simulink model "TrainConvoyMdl"  (R2021b)
settings: Solver=FixedStepAuto  StartTime=0.0  StopTime=500  RelTol=1e-3
undefined symbols (not defined in the file or in its folder): amax_ego, amin_ego, coupling_distance, D_default, DiscIntNeverNeededParam, t_gap, Ts, v0_ego_train_1, v0_ego_train_2, v0_lead_train, v_set, x0_ego_train_1, x0_ego_train_2, x0_lead_train
libraries: simulink x18, rllib x2
settings Model: Creator=The MathWorks, Inc.  LastModifiedBy=danif
settings SolverCC: AlgebraicLoopSolver=TrustRegion
settings DataIOCC: ReturnWorkspaceOutputs=off
settings DebuggingCC: SFMachineParentedDataDiag=warning  ArithmeticOperatorsInVariantConditions=warning
settings SFSimCC: SimUseLocalCustomCode=off
settings RTWCC: RTWUseLocalCustomCode=off
settings CodeAppCC: StateflowObjectComments=on

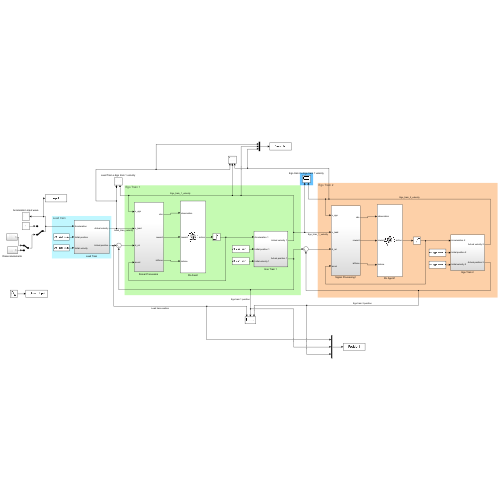
[thumbnail: Simulink's stored preview of the top-level diagram]
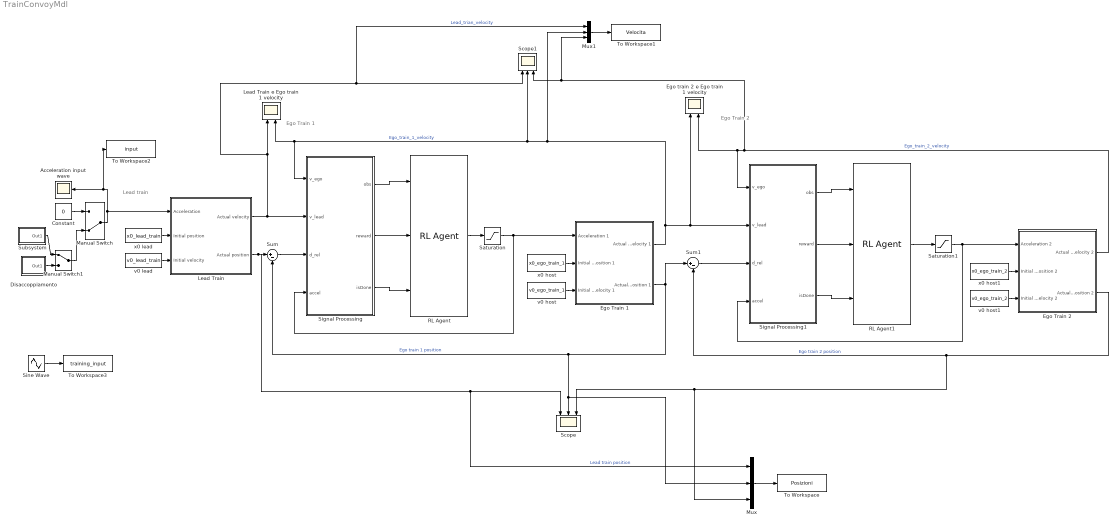
== system TrainConvoyMdl ==
  note: Lead train
  note: Ego Train 1
  note: Ego Train 2
  Acceleration input wave : Scope
  Constant : Constant  Value=0
  Disaccoppiamento : Subsystem
  Ego Train 1 : Subsystem
  Ego Train 2 : Subsystem
  Ego train 2 e Ego train 1 velocity : Scope  NumInputPorts=2
  Lead Train : Subsystem
  Lead Train e Ego train 1 velocity : Scope  NumInputPorts=2
  Manual Switch : ManualSwitch  CurrentSetting=0
  Manual Switch1 : ManualSwitch
  Mux : Mux  Inputs=3
  Mux1 : Mux  Inputs=3
  RL Agent : rllib/RL Agent  Agent=agent  ExternalActionAsInput=off  ProvideCumRwd=off  TreatAsDirectFeedthrough=on
  RL Agent1 : rllib/RL Agent  Agent=agent  ExternalActionAsInput=off  ProvideCumRwd=off  TreatAsDirectFeedthrough=on
  Saturation : Saturate  UpperLimit=amax_ego  LowerLimit=amin_ego
  Saturation1 : Saturate  UpperLimit=amax_ego  LowerLimit=amin_ego-3
  Scope : Scope  NumInputPorts=3
  Scope1 : Scope  NumInputPorts=3
  "Signal Processing " : Subsystem
  Signal Processing1 : Subsystem
  Sine Wave : Sin  Amplitude=0.6  Frequency=0.2  SampleTime=Ts
  Subsystem : Subsystem
  Sum : Sum  Inputs=|+-
  Sum1 : Sum  Inputs=|+-
  To Workspace : ToWorkspace  VariableName=Posizioni  SaveFormat=Timeseries  SampleTime=-1
  To Workspace1 : ToWorkspace  VariableName=Velocita  SaveFormat=Timeseries  SampleTime=-1
  To Workspace2 : ToWorkspace  VariableName=input  SaveFormat=Timeseries  SampleTime=-1
  To Workspace3 : ToWorkspace  VariableName=training_input  SaveFormat=Timeseries  SampleTime=-1
  v0 host : Constant  Value=v0_ego_train_1  SampleTime=Ts
  v0 host1 : Constant  Value=v0_ego_train_2  SampleTime=Ts
  v0 lead : Constant  Value=v0_lead_train  SampleTime=Ts
  x0 host : Constant  Value=x0_ego_train_1  SampleTime=Ts
  x0 host1 : Constant  Value=x0_ego_train_2  SampleTime=Ts
  x0 lead : Constant  Value=x0_lead_train  SampleTime=Ts
  wires:
  x0 lead/1 -> Lead Train/2(Initial position)
  v0 lead/1 -> Lead Train/3(Initial velocity)
  x0 host/1 -> Ego Train 1/2(Initial position 1)
  Ego Train 1/2(Actual position 1) -> Sum1/1, Sum/2, Mux/2, Scope/2  "Ego train 1 position"
  v0 host/1 -> Ego Train 1/3(Initial velocity 1)
  Lead Train/1(Actual velocity) -> "Signal Processing "/2(v_lead), Mux1/1, Scope1/1, Lead Train e Ego train 1 velocity/1  "Lead_trian_velocity"
  "Signal Processing "/2(reward) -> RL Agent/2
  Saturation/1 -> Ego Train 1/1(Acceleration 1), "Signal Processing "/4(accel)
  RL Agent/1 -> Saturation/1
  "Signal Processing "/3(isDone) -> RL Agent/3
  "Signal Processing "/1(obs) -> RL Agent/1
  Sum/1 -> "Signal Processing "/3(d_rel)
  Ego Train 1/1(Actual velocity 1) -> Signal Processing1/2(v_lead), Ego train 2 e Ego train 1 velocity/1, Mux1/2, "Signal Processing "/1(v_ego), Lead Train e Ego train 1 velocity/2, Scope1/2  "Ego_train_1_velocity"
  Ego Train 2/1(Actual velocity 2) -> Signal Processing1/1(v_ego), Ego train 2 e Ego train 1 velocity/2, Mux1/3, Scope1/3  "Ego_train_2_velocity"
  Sum1/1 -> Signal Processing1/3(d_rel)
  Signal Processing1/2(reward) -> RL Agent1/2
  Signal Processing1/1(obs) -> RL Agent1/1
  RL Agent1/1 -> Saturation1/1
  Saturation1/1 -> Ego Train 2/1(Acceleration 2), Signal Processing1/4(accel)
  Signal Processing1/3(isDone) -> RL Agent1/3
  Ego Train 2/2(Actual position 2) -> Mux/3, Scope/3, Sum1/2  "Ego train 2 position"
  v0 host1/1 -> Ego Train 2/3(Initial velocity 2)
  x0 host1/1 -> Ego Train 2/2(Initial position 2)
  Manual Switch/1 -> To Workspace2/1, Acceleration input wave/1, Lead Train/1(Acceleration)
  Constant/1 -> Manual Switch/1
  Lead Train/2(Actual position) -> Mux/1, Scope/1, Sum/1  "Lead train position"
  Disaccoppiamento/1(Out1) -> Manual Switch1/2
  Manual Switch1/1 -> Manual Switch/2
  Subsystem/1(Out1) -> Manual Switch1/1
  Mux/1 -> To Workspace/1
  Mux1/1 -> To Workspace1/1
  Sine Wave/1 -> To Workspace3/1

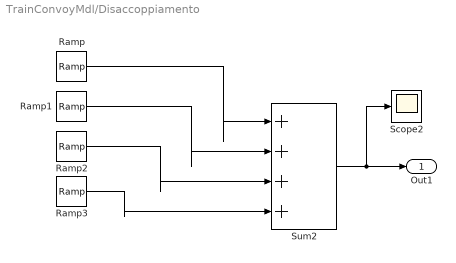
== system TrainConvoyMdl/Disaccoppiamento ==
  Ramp : simulink/Sources/Ramp  slope=0.005  start=70  InitialOutput=0
  Ramp1 : simulink/Sources/Ramp  slope=-0.005  start=130  InitialOutput=0
  Ramp2 : simulink/Sources/Ramp  slope=-0.005  start=260  InitialOutput=0
  Ramp3 : simulink/Sources/Ramp  slope=0.005  start=320  InitialOutput=0
  Scope2 : Scope
  Sum2 : Sum  Inputs=|++++
  Out1 : Outport
  wires:
  Ramp2/1 -> Sum2/3
  Sum2/1 -> Out1/1, Scope2/1
  Ramp1/1 -> Sum2/2
  Ramp3/1 -> Sum2/4
  Ramp/1 -> Sum2/1

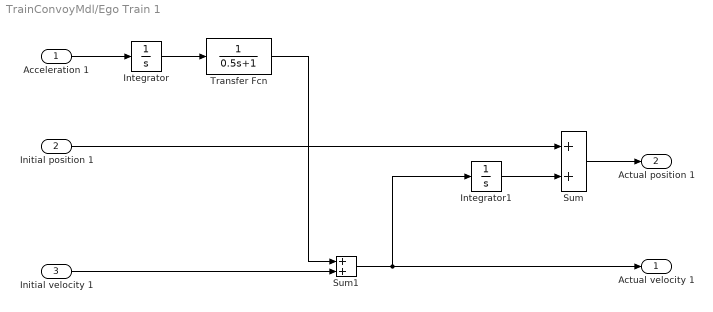
== system TrainConvoyMdl/Ego Train 1 ==
  Acceleration 1 : Inport
  Initial position 1 : Inport  Port=2
  Initial velocity 1 : Inport  Port=3
  Integrator : Integrator
  Integrator1 : Integrator
  Sum : Sum
  Sum1 : Sum
  Transfer Fcn : TransferFcn  Denominator=[0.5 1]
  Actual velocity 1 : Outport  VectorParamsAs1DForOutWhenUnconnected=off
  Actual position 1 : Outport  Port=2  VectorParamsAs1DForOutWhenUnconnected=off
  wires:
  Sum1/1 -> Integrator1/1, Actual velocity 1/1
  Initial velocity 1/1 -> Sum1/2
  Sum/1 -> Actual position 1/1
  Transfer Fcn/1 -> Sum1/1
  Integrator/1 -> Transfer Fcn/1
  Acceleration 1/1 -> Integrator/1
  Initial position 1/1 -> Sum/1
  Integrator1/1 -> Sum/2

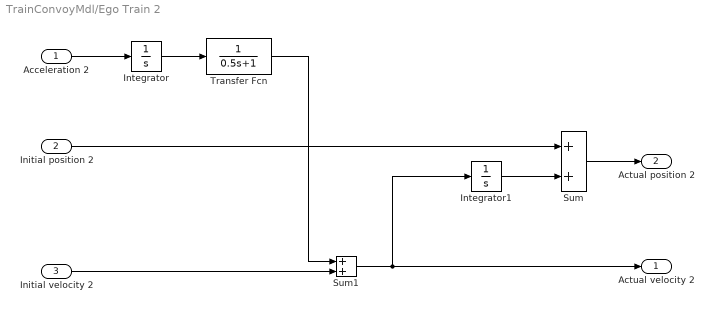
== system TrainConvoyMdl/Ego Train 2 ==
  Acceleration 2 : Inport
  Initial position 2 : Inport  Port=2
  Initial velocity 2 : Inport  Port=3
  Integrator : Integrator
  Integrator1 : Integrator
  Sum : Sum
  Sum1 : Sum
  Transfer Fcn : TransferFcn  Denominator=[0.5 1]
  Actual velocity 2 : Outport  VectorParamsAs1DForOutWhenUnconnected=off
  Actual position 2 : Outport  Port=2  VectorParamsAs1DForOutWhenUnconnected=off
  wires:
  Sum1/1 -> Integrator1/1, Actual velocity 2/1
  Initial velocity 2/1 -> Sum1/2
  Sum/1 -> Actual position 2/1
  Transfer Fcn/1 -> Sum1/1
  Integrator/1 -> Transfer Fcn/1
  Acceleration 2/1 -> Integrator/1
  Initial position 2/1 -> Sum/1
  Integrator1/1 -> Sum/2

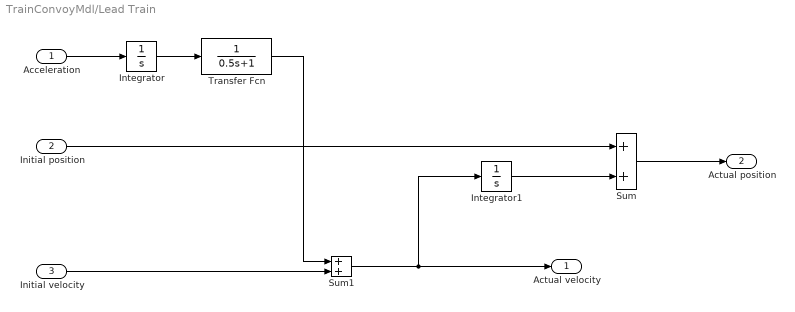
== system TrainConvoyMdl/Lead Train ==
  Acceleration : Inport
  Initial position : Inport  Port=2
  Initial velocity : Inport  Port=3
  Integrator : Integrator
  Integrator1 : Integrator
  Sum : Sum
  Sum1 : Sum
  Transfer Fcn : TransferFcn  Denominator=[0.5 1]
  Actual velocity : Outport  VectorParamsAs1DForOutWhenUnconnected=off
  Actual position : Outport  Port=2  VectorParamsAs1DForOutWhenUnconnected=off
  wires:
  Transfer Fcn/1 -> Sum1/1
  Initial velocity/1 -> Sum1/2
  Sum/1 -> Actual position/1
  Integrator/1 -> Transfer Fcn/1
  Sum1/1 -> Integrator1/1, Actual velocity/1
  Acceleration/1 -> Integrator/1
  Initial position/1 -> Sum/1
  Integrator1/1 -> Sum/2

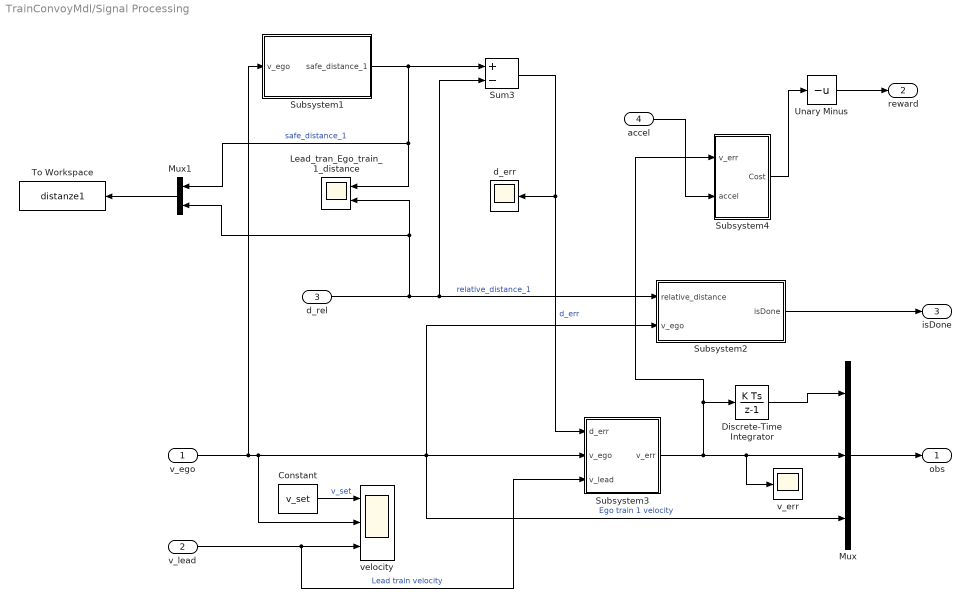
== system TrainConvoyMdl/Signal Processing  ==
  v_ego : Inport
  v_lead : Inport  Port=2
  d_rel : Inport  Port=3
  accel : Inport  Port=4
  Constant : Constant  Value=v_set
  Discrete-Time Integrator : DiscreteIntegrator  SampleTime=-1  ICPrevOutput=DiscIntNeverNeededParam  ICPrevScaledInput=DiscIntNeverNeededParam
  Lead_tran_Ego_train_1_distance : Scope  NumInputPorts=2
  Mux : Mux  Inputs=3
  Mux1 : Mux  Inputs=2
  Subsystem1 : Subsystem
  Subsystem2 : Subsystem
  Subsystem3 : Subsystem
  Subsystem4 : Subsystem
  Sum3 : Sum  Inputs=+-
  To Workspace : ToWorkspace  VariableName=distanze1  SaveFormat=Timeseries  SampleTime=-1
  Unary Minus : UnaryMinus
  d_err : Scope
  v_err : Scope
  velocity : Scope  NumInputPorts=3
  obs : Outport  VectorParamsAs1DForOutWhenUnconnected=off
  reward : Outport  Port=2  VectorParamsAs1DForOutWhenUnconnected=off
  isDone : Outport  Port=3  VectorParamsAs1DForOutWhenUnconnected=off
  wires:
  Constant/1 -> velocity/1  "v_set"
  v_lead/1 -> velocity/3, Subsystem3/3(v_lead)  "Lead train velocity"
  Mux/1 -> obs/1
  v_ego/1 -> velocity/2, Subsystem3/2(v_ego), Mux/3, Subsystem2/2(v_ego), Subsystem1/1(v_ego)  "Ego train 1 velocity"
  d_rel/1 -> Subsystem2/1(relative_distance), Sum3/2, Mux1/2, Lead_tran_Ego_train_1_distance/2  "relative_distance_1"
  Subsystem4/1(Cost) -> Unary Minus/1
  Unary Minus/1 -> reward/1
  Sum3/1 -> Subsystem3/1(d_err), d_err/1  "d_err"
  Subsystem1/1(safe_distance_1) -> Mux1/1, Lead_tran_Ego_train_1_distance/1, Sum3/1  "safe_distance_1"
  accel/1 -> Subsystem4/2(accel)
  Subsystem2/1(isDone) -> isDone/1
  Subsystem3/1(v_err) -> Subsystem4/1(v_err), Discrete-Time Integrator/1, v_err/1, Mux/2
  Discrete-Time Integrator/1 -> Mux/1
  Mux1/1 -> To Workspace/1

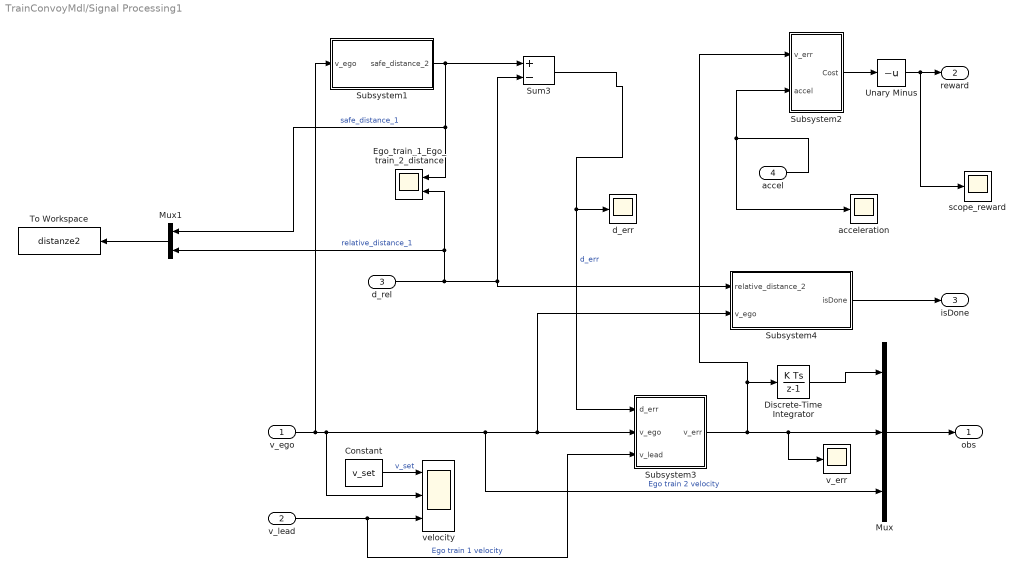
== system TrainConvoyMdl/Signal Processing1 ==
  v_ego : Inport
  v_lead : Inport  Port=2
  d_rel : Inport  Port=3
  accel : Inport  Port=4
  Constant : Constant  Value=v_set
  Discrete-Time Integrator : DiscreteIntegrator  SampleTime=-1  ICPrevOutput=DiscIntNeverNeededParam  ICPrevScaledInput=DiscIntNeverNeededParam
  Ego_train_1_Ego_train_2_distance : Scope  NumInputPorts=2
  Mux : Mux  Inputs=3
  Mux1 : Mux  Inputs=2
  Subsystem1 : Subsystem
  Subsystem2 : Subsystem
  Subsystem3 : Subsystem
  Subsystem4 : Subsystem
  Sum3 : Sum  Inputs=+-
  To Workspace : ToWorkspace  VariableName=distanze2  SaveFormat=Timeseries  SampleTime=-1
  Unary Minus : UnaryMinus
  acceleration : Scope
  d_err : Scope
  scope_reward : Scope
  v_err : Scope
  velocity : Scope  NumInputPorts=3
  obs : Outport  VectorParamsAs1DForOutWhenUnconnected=off
  reward : Outport  Port=2  VectorParamsAs1DForOutWhenUnconnected=off
  isDone : Outport  Port=3  VectorParamsAs1DForOutWhenUnconnected=off
  wires:
  Constant/1 -> velocity/1  "v_set"
  v_lead/1 -> velocity/3, Subsystem3/3(v_lead)  "Ego train 1 velocity"
  Mux/1 -> obs/1
  v_ego/1 -> velocity/2, Subsystem4/2(v_ego), Subsystem3/2(v_ego), Mux/3, Subsystem1/1(v_ego)  "Ego train 2 velocity"
  Subsystem2/1(Cost) -> Unary Minus/1
  Sum3/1 -> d_err/1, Subsystem3/1(d_err)  "d_err"
  accel/1 -> Subsystem2/2(accel), acceleration/1
  Subsystem4/1(isDone) -> isDone/1
  Subsystem3/1(v_err) -> Subsystem2/1(v_err), Discrete-Time Integrator/1, v_err/1, Mux/2
  Discrete-Time Integrator/1 -> Mux/1
  Unary Minus/1 -> scope_reward/1, reward/1
  d_rel/1 -> Subsystem4/1(relative_distance_2), Sum3/2, Ego_train_1_Ego_train_2_distance/2, Mux1/2  "relative_distance_1"
  Mux1/1 -> To Workspace/1
  Subsystem1/1(safe_distance_2) -> Mux1/1, Ego_train_1_Ego_train_2_distance/1, Sum3/1  "safe_distance_1"

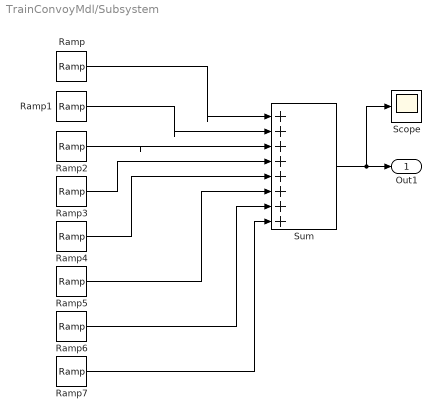
== system TrainConvoyMdl/Subsystem ==
  Ramp : simulink/Sources/Ramp  slope=0.005  start=70  InitialOutput=0
  Ramp1 : simulink/Sources/Ramp  slope=-0.005  start=110  InitialOutput=0
  Ramp2 : simulink/Sources/Ramp  slope=-0.005  start=140  InitialOutput=0
  Ramp3 : simulink/Sources/Ramp  slope=0.005  start=180  InitialOutput=0
  Ramp4 : simulink/Sources/Ramp  slope=-0.005  start=230  InitialOutput=0
  Ramp5 : simulink/Sources/Ramp  slope=0.005  start=280  InitialOutput=0
  Ramp6 : simulink/Sources/Ramp  slope=0.005  start=320  InitialOutput=0
  Ramp7 : simulink/Sources/Ramp  slope=-0.005  start=370  InitialOutput=0
  Scope : Scope
  Sum : Sum  Inputs=|++++++++
  Out1 : Outport
  wires:
  Ramp/1 -> Sum/1
  Ramp2/1 -> Sum/3
  Ramp1/1 -> Sum/2
  Ramp3/1 -> Sum/4
  Sum/1 -> Scope/1, Out1/1
  Ramp4/1 -> Sum/5
  Ramp5/1 -> Sum/6
  Ramp6/1 -> Sum/7
  Ramp7/1 -> Sum/8

== system TrainConvoyMdl/Signal Processing /Subsystem1 ==
  v_ego : Inport
  Default Spacing : Constant  Value=D_default  SampleTime=Ts
  Product : Product
  Sum2 : Sum
  Time Gap : Constant  Value=t_gap  SampleTime=Ts
  safe_distance_1 : Outport  VectorParamsAs1DForOutWhenUnconnected=off
  wires:
  Sum2/1 -> safe_distance_1/1
  Time Gap/1 -> Product/2
  Default Spacing/1 -> Sum2/1
  v_ego/1 -> Product/1
  Product/1 -> Sum2/2

== system TrainConvoyMdl/Signal Processing /Subsystem2 ==
  relative_distance : Inport
  v_ego : Inport  Port=2
  Logical Operator : Logic  Operator=OR  AllPortsSameDT=off  OutDataTypeStr=boolean
  Relative Distance : simulink/Logic and Bit Operations/Compare To Constant  relop=<  const=0  OutDataTypeStr=boolean
  Velocity : simulink/Logic and Bit Operations/Compare To Constant  relop=<  const=0  OutDataTypeStr=boolean
  isDone : Outport  VectorParamsAs1DForOutWhenUnconnected=off
  wires:
  Velocity/1 -> Logical Operator/2
  Relative Distance/1 -> Logical Operator/1
  Logical Operator/1 -> isDone/1
  v_ego/1 -> Velocity/1
  relative_distance/1 -> Relative Distance/1

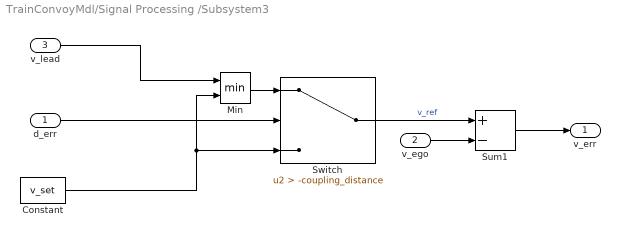
== system TrainConvoyMdl/Signal Processing /Subsystem3 ==
  d_err : Inport
  v_ego : Inport  Port=2
  v_lead : Inport  Port=3
  Constant : Constant  Value=v_set
  Min : MinMax  Inputs=2
  Sum1 : Sum  Inputs=+-
  Switch : Switch  Criteria=u2 > Threshold  Threshold=-coupling_distance
  v_err : Outport  VectorParamsAs1DForOutWhenUnconnected=off
  wires:
  Sum1/1 -> v_err/1
  v_ego/1 -> Sum1/2
  d_err/1 -> Switch/2
  Constant/1 -> Min/2, Switch/3
  Min/1 -> Switch/1
  v_lead/1 -> Min/1
  Switch/1 -> Sum1/1  "v_ref"

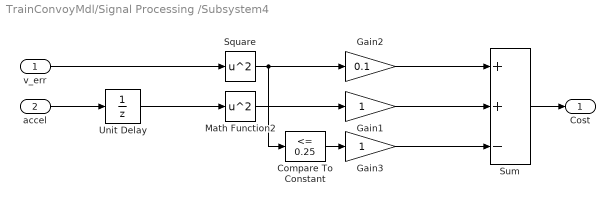
== system TrainConvoyMdl/Signal Processing /Subsystem4 ==
  v_err : Inport
  accel : Inport  Port=2
  Compare To Constant : simulink/Logic and Bit Operations/Compare To Constant  relop=<=  const=0.25  OutDataTypeStr=boolean
  Gain1 : Gain
  Gain2 : Gain  Gain=0.1
  Gain3 : Gain
  Math Function2 : Math  Operator=square  SignedPower=on  SaturateOnIntegerOverflow=on
  Square : Math  Operator=square  SignedPower=on  SaturateOnIntegerOverflow=on
  Sum : Sum  Inputs=++-
  Unit Delay : UnitDelay  SampleTime=-1  HasFrameUpgradeWarning=on
  Cost : Outport  VectorParamsAs1DForOutWhenUnconnected=off
  wires:
  v_err/1 -> Square/1
  Math Function2/1 -> Gain1/1
  accel/1 -> Unit Delay/1
  Sum/1 -> Cost/1
  Square/1 -> Compare To Constant/1, Gain2/1
  Unit Delay/1 -> Math Function2/1
  Gain2/1 -> Sum/1
  Gain1/1 -> Sum/2
  Compare To Constant/1 -> Gain3/1
  Gain3/1 -> Sum/3

== system TrainConvoyMdl/Signal Processing1/Subsystem1 ==
  v_ego : Inport
  Default Spacing : Constant  Value=D_default  SampleTime=Ts
  Product : Product
  Sum2 : Sum
  Time Gap : Constant  Value=t_gap  SampleTime=Ts
  safe_distance_2 : Outport  VectorParamsAs1DForOutWhenUnconnected=off
  wires:
  Sum2/1 -> safe_distance_2/1
  Time Gap/1 -> Product/2
  Default Spacing/1 -> Sum2/1
  v_ego/1 -> Product/1
  Product/1 -> Sum2/2

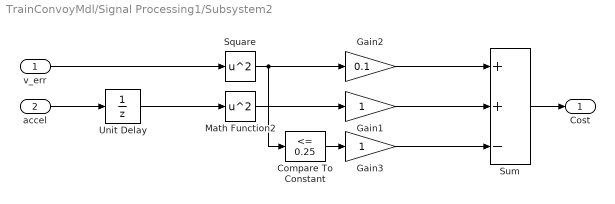
== system TrainConvoyMdl/Signal Processing1/Subsystem2 ==
  v_err : Inport
  accel : Inport  Port=2
  Compare To Constant : simulink/Logic and Bit Operations/Compare To Constant  relop=<=  const=0.25  OutDataTypeStr=boolean
  Gain1 : Gain
  Gain2 : Gain  Gain=0.1
  Gain3 : Gain
  Math Function2 : Math  Operator=square  SignedPower=on  SaturateOnIntegerOverflow=on
  Square : Math  Operator=square  SignedPower=on  SaturateOnIntegerOverflow=on
  Sum : Sum  Inputs=++-
  Unit Delay : UnitDelay  SampleTime=-1  HasFrameUpgradeWarning=on
  Cost : Outport  VectorParamsAs1DForOutWhenUnconnected=off
  wires:
  v_err/1 -> Square/1
  Math Function2/1 -> Gain1/1
  accel/1 -> Unit Delay/1
  Sum/1 -> Cost/1
  Square/1 -> Compare To Constant/1, Gain2/1
  Unit Delay/1 -> Math Function2/1
  Gain2/1 -> Sum/1
  Gain1/1 -> Sum/2
  Compare To Constant/1 -> Gain3/1
  Gain3/1 -> Sum/3

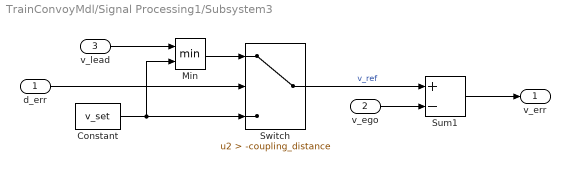
== system TrainConvoyMdl/Signal Processing1/Subsystem3 ==
  d_err : Inport
  v_ego : Inport  Port=2
  v_lead : Inport  Port=3
  Constant : Constant  Value=v_set
  Min : MinMax  Inputs=2
  Sum1 : Sum  Inputs=+-
  Switch : Switch  Criteria=u2 > Threshold  Threshold=-coupling_distance
  v_err : Outport  VectorParamsAs1DForOutWhenUnconnected=off
  wires:
  Sum1/1 -> v_err/1
  v_ego/1 -> Sum1/2
  d_err/1 -> Switch/2
  Constant/1 -> Min/2, Switch/3
  Min/1 -> Switch/1
  v_lead/1 -> Min/1
  Switch/1 -> Sum1/1  "v_ref"

== system TrainConvoyMdl/Signal Processing1/Subsystem4 ==
  relative_distance_2 : Inport
  v_ego : Inport  Port=2
  Logical Operator : Logic  Operator=OR  AllPortsSameDT=off  OutDataTypeStr=boolean
  Relative Distance : simulink/Logic and Bit Operations/Compare To Constant  relop=<  const=0  OutDataTypeStr=boolean
  Velocity : simulink/Logic and Bit Operations/Compare To Constant  relop=<  const=0  OutDataTypeStr=boolean
  isDone : Outport  VectorParamsAs1DForOutWhenUnconnected=off
  wires:
  Velocity/1 -> Logical Operator/2
  Relative Distance/1 -> Logical Operator/1
  Logical Operator/1 -> isDone/1
  v_ego/1 -> Velocity/1
  relative_distance_2/1 -> Relative Distance/1
